simulink model "min_state_observer"  (R2025b)
settings: Solver=VariableStepAuto  StartTime=0.0  StopTime=20  RelTol=1e-3
values from neighbouring files (symbols this model uses):
  A = [0 1 0 0 ... (first row only)    [untitled2.m]    (also in untitled3.m)
  A_hat = A_bb - Ke*A_ab    [untitled2.m]
  B = [0; 0; 0; 1/m2]    [untitled2.m]    (also in untitled3.m = [0;1/m1;0;0])
  B_hat = A_hat*Ke + A_ba - Ke*A_aa    [untitled2.m]
  C = [1 0 0 0]    [untitled2.m]
  C_hat = [zeros(1, 3) ... (first row only)    [untitled2.m]
  D_hat = [1 ... (first row only)    [untitled2.m]
  F_hat = B_b - Ke*B_a    [untitled2.m]
  Ke = place(A_bb', A_ab', p_o)'    [untitled2.m]
  x0 = [1; 0; -1; 0]    [untitled2.m]
  z0 = [2; 1.5; 1]    [untitled2.m]
settings Model: Creator=abhi  LastModifiedBy=Abhi

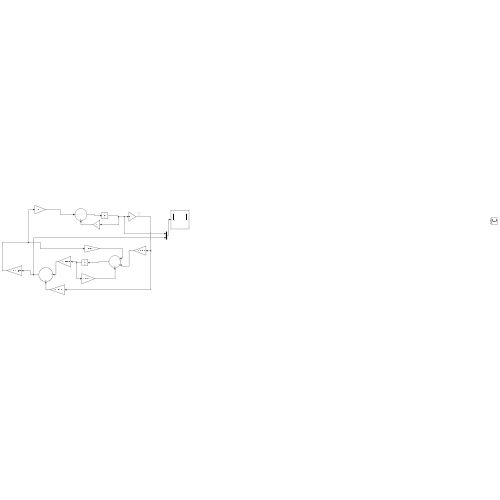
[thumbnail: Simulink's stored preview of the top-level diagram]
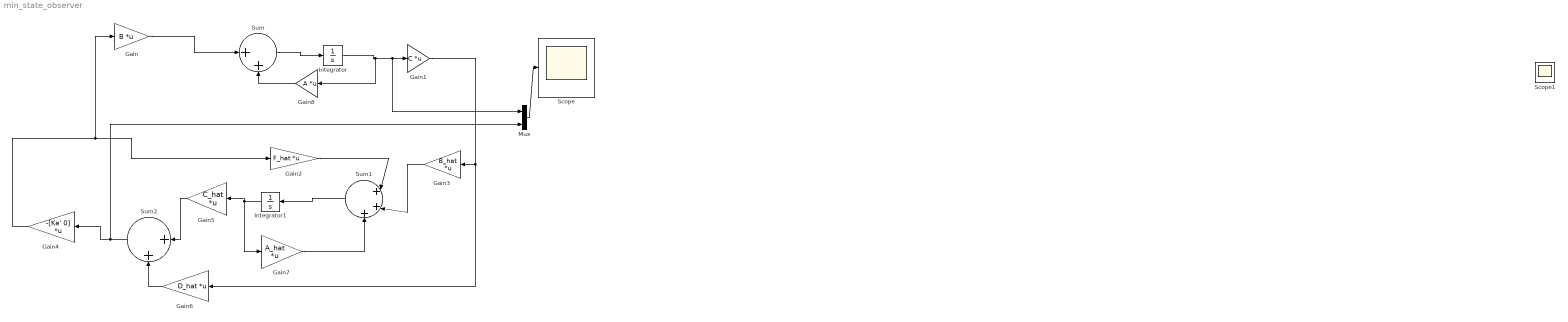
== system min_state_observer ==
  Gain : Gain  Gain=B  Multiplication=Matrix(K*u)
  Gain1 : Gain  Gain=C  Multiplication=Matrix(K*u)
  Gain2 : Gain  Gain=F_hat  Multiplication=Matrix(K*u)
  Gain3 : Gain  Gain=B_hat  Multiplication=Matrix(K*u)
  Gain4 : Gain  Gain=-[Ke' 0]  Multiplication=Matrix(K*u)
  Gain5 : Gain  Gain=C_hat  Multiplication=Matrix(K*u)
  Gain6 : Gain  Gain=D_hat  Multiplication=Matrix(K*u)
  Gain7 : Gain  Gain=A_hat  Multiplication=Matrix(K*u)
  Gain8 : Gain  Gain=A  Multiplication=Matrix(K*u)
  Integrator : Integrator  InitialCondition=x0
  Integrator1 : Integrator  InitialCondition=z0
  Mux : Mux  Inputs=2
  Scope : Scope
      settings: ActiveDisplayYMinimum=-1.4589097055868172  ActiveDisplayYMaximum=1.5082704382374088
  Scope1 : Scope  NumInputPorts=2
      settings: ActiveDisplayYMinimum=-1.16819116268996  ActiveDisplayYMaximum=1.1667330676781473
  Sum : Sum  Inputs=|++
  Sum1 : Sum  Inputs=|+++
  Sum2 : Sum  Inputs=|++
  wires:
  Integrator/1 -> Gain8/1, Mux/1, Gain1/1
  Gain3/1 -> Sum1/2
  Gain2/1 -> Sum1/1
  Gain6/1 -> Sum2/2
  Gain5/1 -> Sum2/1
  Integrator1/1 -> Gain5/1, Gain7/1
  Gain7/1 -> Sum1/3
  Sum1/1 -> Integrator1/1
  Sum2/1 -> Mux/2, Gain4/1
  Gain4/1 -> Gain2/1, Gain/1
  Gain1/1 -> Gain6/1, Gain3/1
  Sum/1 -> Integrator/1
  Gain8/1 -> Sum/2
  Gain/1 -> Sum/1
  Mux/1 -> Scope/1
